simulink model "Bruening_4t_showshuffle"  (R2015a)
settings: Solver=ode4  SolverMode=MultiTasking  StartTime=0.0  StopTime=inf  FixedStep=BKIN_STEP_TIME  RelTol=1e-3
StartFcn:
  |  warndlg('Dexterit-E models cannot run under simulation. Please compile your model and run it from within Dexterit-E.');set_param(bdroot,'SimulationCommand','stop')
model workspace (MAT data in the model file):
  BKIN_STEP_TIME = 0.00025
  col_x = 1
  col_y = 2
  E_TARGET_ON = 3
  E_HOLD_AT_TARGET = 5
  LOGICAL_RADIUS = 4
  START_TARGET_COL = 1
  END_TARGET_COL = 2
  ROTATION_CENTER = 5
  WAIT_AT_1stTARGET_COL = 7
  MAXREACHTIME_COL = 8
  DELAY_POSTTRIAL_COL = 9
  E_STAY_CENTER = 2
  VISUAL_RADIUS = 3
  COLOR = 5
  ALTCOLOR = 6
  STROKECOLOUR = 7
  STROKEWIDTH = 9
  TARGET_EGG = 6
  LABEL_TEXT = 12
  LABEL_COLOUR = 13
  LABEL_HEIGHT = 14
  TEXT_DISPLAY_TARGET = 10
  ALTSTROKECOLOUR = 8
  SEGMENT_COUNT = 11
  E_TARGET_MISS = 6
  END_X = 10
  END_Y = 11
  E_LEFT_RING = 4
  E_START_BLOCK = 10
  BKIN_KINEMATIC_FRAME_SIZE = 400
  E_NO_EVENT = 1
  TARGET_IN_USE = 3
  R_PROB = 4
  E_R_TARG1 = 7
  E_M_TARG1 = 12
  E_R_TARG2 = 8
  E_M_TARG2 = 13
  E_R_TARG3 = 9
  E_M_TARG3 = 14
  E_R_TARG4 = 11
  E_M_TARG4 = 15
  WAIT_TIME = 12
  TONE_DURATION = 13
  FLASH_INTER = 14
  FLASH_NUM = 15
  BREAK_T1 = 16
  BREAK_T2 = 17
  ALTVISUAL_RADIUS = 15
  ALTCOLOR2 = 16
undefined symbols (not defined in the file or in its folder): slselsubs
libraries: Video x15, simulink x12, xpcrtudplib x12, xpcutilitieslib x10, xpcobsoletelib x8, ethercat x2, General x2, slrtlib x2, KINARM_general x1
(part 2 of 6)

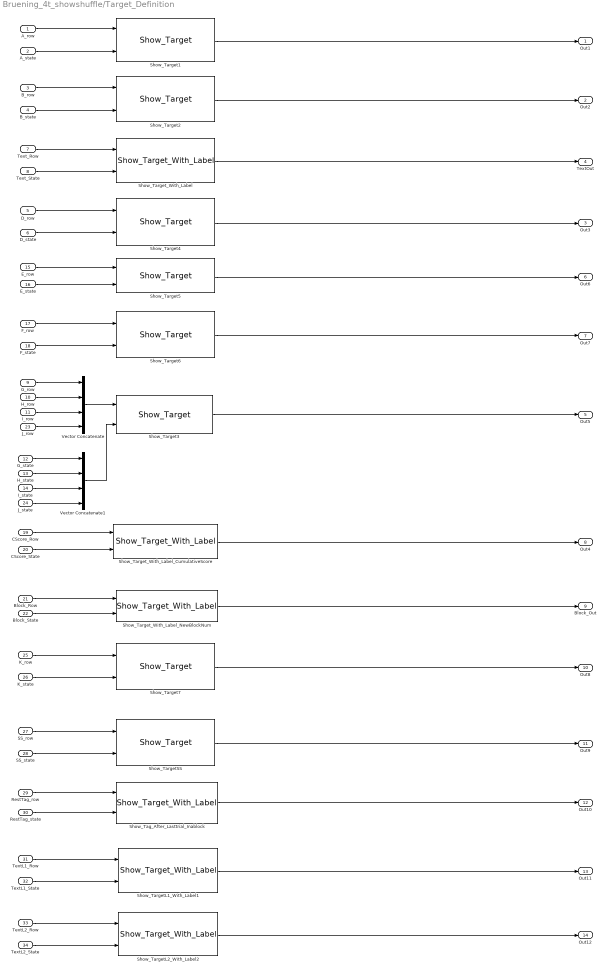
== system Bruening_4t_showshuffle/Target_Definition  ==
  A_row : Inport
  A_state : Inport  Port=2
  B_row : Inport  Port=3
  B_state : Inport  Port=4
  D_row : Inport  Port=5
  D_state : Inport  Port=6
  Text_Row : Inport  Port=7
  Text_State : Inport  Port=8
  G_row : Inport  Port=9
  H_row : Inport  Port=10
  I_row : Inport  Port=11
  G_state : Inport  Port=12
  H_state : Inport  Port=13
  I_state : Inport  Port=14
  E_row : Inport  Port=15
  E_state : Inport  Port=16
  F_row : Inport  Port=17
  F_state : Inport  Port=18
  CScore_Row : Inport  Port=19
  CScore_State : Inport  Port=20
  Block_Row : Inport  Port=21
  Block_State : Inport  Port=22
  J_row : Inport  Port=23
  J_state : Inport  Port=24
  K_row : Inport  Port=25
  K_state : Inport  Port=26
  SS_row : Inport  Port=27
  SS_state : Inport  Port=28
  RestTag_row : Inport  Port=29
  RestTag_state : Inport  Port=30
  TextL1_Row : Inport  Port=31
  TextL1_State : Inport  Port=32
  TextL2_Row : Inport  Port=33
  TextL2_State : Inport  Port=34
  Show_Tag_After_Lasttrial_Inablock : Video/Show_Target_With_Label  target_type=Circle  num_states=1  attribcol1=[0 5 0 VISUAL_RADIUS LABEL_TEXT LABEL_COLOUR LABEL_HEIGHT]  attribcol2=[6 6 0 3 0 0 0]  attribcol3=[0 0 0 0 0 0 0]  attribcol4=[0 0 0 0 0 0 0]  attribcol5=[0 0 24 0 0 0 0]  stateindices_padding=[0 0 0 0;0 0 0 0;0 0 0 0;0 0 0 0;0 0 0 0]  source=dialog  opacity=100  target_display=Both subject and operator displays
  Show_Target1 : Video/Show_Target  target_type=Circle  num_states=2  attribcol1=[COLOR 0 0 VISUAL_RADIUS]  attribcol2=[ALTCOLOR 0 0 VISUAL_RADIUS]  attribcol3=[0 0 0 0]  attribcol4=[0 0 0 0]  attribcol5=[0 0 24 0]  stateindices_padding=[0 0 0 0 0 0 0;0 0 0 0 0 0 0;0 0 0 0 0 0 0;0 0 0 0 0 0 0;0 0 0 0 0 0 0]  source=dialog  opacity=100  target_display=Both subject and operator displays  num_col=4
  Show_Target2 : Video/Show_Target  target_type=Circle  num_states=2  attribcol1=[COLOR STROKECOLOUR STROKEWIDTH VISUAL_RADIUS]  attribcol2=[COLOR ALTSTROKECOLOUR STROKEWIDTH VISUAL_RADIUS]  attribcol3=[0 0 0 0]  attribcol4=[0 0 0 0]  attribcol5=[0 0 24 0]  stateindices_padding=[0 0 0 0 0 0 0;0 0 0 0 0 0 0;0 0 0 0 0 0 0;0 0 0 0 0 0 0;0 0 0 0 0 0 0]  source=dialog  opacity=100  target_display=Both subject and operator displays  num_col=4
  Show_Target3 : Video/Show_Target  target_type=Line  num_states=2  attribcol1=[0 STROKECOLOUR STROKEWIDTH END_X END_Y]  attribcol2=[0 ALTSTROKECOLOUR STROKEWIDTH END_X END_Y]  attribcol3=[0 0 0 0 0]  attribcol4=[0 0 0 0 0]  attribcol5=[0 0 24 0 0]  stateindices_padding=[0 0 0 0 0 0;0 0 0 0 0 0;0 0 0 0 0 0;0 0 0 0 0 0;0 0 0 0 0 0]  source=dialog  opacity=100  target_display=Both subject and operator displays  num_col=5
  Show_Target4 : Video/Show_Target  target_type=Circle  num_states=3  attribcol1=[COLOR STROKECOLOUR STROKEWIDTH VISUAL_RADIUS]  attribcol2=[ALTCOLOR STROKECOLOUR STROKEWIDTH ALTVISUAL_RADIUS]  attribcol3=[ALTCOLOR2 STROKECOLOUR STROKEWIDTH VISUAL_RADIUS]  attribcol4=[0 0 0 0]  attribcol5=[0 0 24 0]  stateindices_padding=[0 0 0 0 0 0 0;0 0 0 0 0 0 0;0 0 0 0 0 0 0;0 0 0 0 0 0 0;0 0 0 0 0 0 0]  source=dialog  opacity=100  target_display=Both subject and operator displays  num_col=4
  Show_Target5 : Video/Show_Target  target_type=Circle  num_states=3  attribcol1=[COLOR STROKECOLOUR STROKEWIDTH VISUAL_RADIUS]  attribcol2=[ALTCOLOR ALTSTROKECOLOUR STROKEWIDTH ALTVISUAL_RADIUS]  attribcol3=[ALTCOLOR2 STROKECOLOUR STROKEWIDTH VISUAL_RADIUS]  attribcol4=[0 0 0 0]  attribcol5=[0 0 24 0]  stateindices_padding=[0 0 0 0 0 0 0;0 0 0 0 0 0 0;0 0 0 0 0 0 0;0 0 0 0 0 0 0;0 0 0 0 0 0 0]  source=dialog  opacity=100  target_display=Both subject and operator displays  num_col=4
  Show_Target6 : Video/Show_Target  target_type=Circle  num_states=3  attribcol1=[COLOR STROKECOLOUR STROKEWIDTH VISUAL_RADIUS]  attribcol2=[ALTCOLOR ALTSTROKECOLOUR STROKEWIDTH ALTVISUAL_RADIUS]  attribcol3=[ALTCOLOR2 STROKECOLOUR STROKEWIDTH VISUAL_RADIUS]  attribcol4=[0 0 0 0]  attribcol5=[0 0 24 0]  stateindices_padding=[0 0 0 0 0 0 0;0 0 0 0 0 0 0;0 0 0 0 0 0 0;0 0 0 0 0 0 0;0 0 0 0 0 0 0]  source=dialog  opacity=100  target_display=Both subject and operator displays  num_col=4
  Show_Target7 : Video/Show_Target  target_type=Circle  num_states=3  attribcol1=[COLOR STROKECOLOUR STROKEWIDTH VISUAL_RADIUS]  attribcol2=[ALTCOLOR ALTSTROKECOLOUR STROKEWIDTH ALTVISUAL_RADIUS]  attribcol3=[ALTCOLOR2 STROKECOLOUR STROKEWIDTH VISUAL_RADIUS]  attribcol4=[0 0 0 0]  attribcol5=[0 0 24 0]  stateindices_padding=[0 0 0 0 0 0 0;0 0 0 0 0 0 0;0 0 0 0 0 0 0;0 0 0 0 0 0 0;0 0 0 0 0 0 0]  source=dialog  opacity=100  target_display=Both subject and operator displays  num_col=4
  Show_TargetL1_With_Label1 : Video/Show_Target_With_Label  target_type=Circle  num_states=1  attribcol1=[0 5 0 VISUAL_RADIUS LABEL_TEXT LABEL_COLOUR LABEL_HEIGHT]  attribcol2=[0 6 0 VISUAL_RADIUS LABEL_TEXT LABEL_COLOUR LABEL_HEIGHT]  attribcol3=[0 0 0 0 0 0 0]  attribcol4=[0 0 0 0 0 0 0]  attribcol5=[0 0 24 0 0 0 0]  stateindices_padding=[0 0 0 0;0 0 0 0;0 0 0 0;0 0 0 0;0 0 0 0]  source=dialog  opacity=100  target_display=Both subject and operator displays
  Show_TargetL2_With_Label2 : Video/Show_Target_With_Label  target_type=Circle  num_states=1  attribcol1=[0 5 0 VISUAL_RADIUS LABEL_TEXT LABEL_COLOUR LABEL_HEIGHT]  attribcol2=[0 6 0 VISUAL_RADIUS LABEL_TEXT LABEL_COLOUR LABEL_HEIGHT]  attribcol3=[0 0 0 0 0 0 0]  attribcol4=[0 0 0 0 0 0 0]  attribcol5=[0 0 24 0 0 0 0]  stateindices_padding=[0 0 0 0;0 0 0 0;0 0 0 0;0 0 0 0;0 0 0 0]  source=dialog  opacity=100  target_display=Both subject and operator displays
  Show_TargetSS : Video/Show_Target  target_type=Circle  num_states=2  attribcol1=[COLOR STROKECOLOUR STROKEWIDTH VISUAL_RADIUS]  attribcol2=[ALTCOLOR ALTSTROKECOLOUR STROKEWIDTH VISUAL_RADIUS]  attribcol3=[0 0 0 0]  attribcol4=[0 0 0 0]  attribcol5=[0 0 24 0]  stateindices_padding=[0 0 0 0 0 0 0;0 0 0 0 0 0 0;0 0 0 0 0 0 0;0 0 0 0 0 0 0;0 0 0 0 0 0 0]  source=dialog  opacity=100  target_display=Both subject and operator displays  num_col=4
  Show_Target_With_Label : Video/Show_Target_With_Label  target_type=Circle  num_states=1  attribcol1=[0 5 0 VISUAL_RADIUS LABEL_TEXT LABEL_COLOUR LABEL_HEIGHT]  attribcol2=[0 6 0 VISUAL_RADIUS LABEL_TEXT LABEL_COLOUR LABEL_HEIGHT]  attribcol3=[0 0 0 0 0 0 0]  attribcol4=[0 0 0 0 0 0 0]  attribcol5=[0 0 24 0 0 0 0]  stateindices_padding=[0 0 0 0;0 0 0 0;0 0 0 0;0 0 0 0;0 0 0 0]  source=dialog  opacity=100  target_display=Both subject and operator displays
  Show_Target_With_Label_CumulativeScore : Video/Show_Target_With_Label  target_type=Circle  num_states=1  attribcol1=[0 5 0 VISUAL_RADIUS LABEL_TEXT LABEL_COLOUR LABEL_HEIGHT]  attribcol2=[6 6 0 3 0 0 0]  attribcol3=[0 0 0 0 0 0 0]  attribcol4=[0 0 0 0 0 0 0]  attribcol5=[0 0 24 0 0 0 0]  stateindices_padding=[0 0 0 0;0 0 0 0;0 0 0 0;0 0 0 0;0 0 0 0]  source=dialog  opacity=100  target_display=Both subject and operator displays
  Show_Target_With_Label_NewBlockNum : Video/Show_Target_With_Label  target_type=Circle  num_states=1  attribcol1=[0 5 0 VISUAL_RADIUS LABEL_TEXT LABEL_COLOUR LABEL_HEIGHT]  attribcol2=[6 6 0 3 0 0 0]  attribcol3=[0 0 0 0 0 0 0]  attribcol4=[0 0 0 0 0 0 0]  attribcol5=[0 0 24 0 0 0 0]  stateindices_padding=[0 0 0 0;0 0 0 0;0 0 0 0;0 0 0 0;0 0 0 0]  source=dialog  opacity=100  target_display=Both subject and operator displays
  Vector Concatenate : Concatenate  NumInputs=4  Mode=Multidimensional array
  Vector Concatenate1 : Concatenate  NumInputs=4  Mode=Multidimensional array
  Out1 : Outport
  Out2 : Outport  Port=2
  Out3 : Outport  Port=3
  TextOut : Outport  Port=4
  Out5 : Outport  Port=5
  Out6 : Outport  Port=6
  Out7 : Outport  Port=7
  Out4 : Outport  Port=8
  Block_Out : Outport  Port=9
  Out8 : Outport  Port=10
  Out9 : Outport  Port=11
  Out10 : Outport  Port=12
  Out11 : Outport  Port=13
  Out12 : Outport  Port=14
  wires:
  Show_Target1/1 -> Out1/1
  A_state/1 -> Show_Target1/2
  A_row/1 -> Show_Target1/1
  Text_Row/1 -> Show_Target_With_Label/1
  Text_State/1 -> Show_Target_With_Label/2
  Show_Target_With_Label/1 -> TextOut/1
  G_row/1 -> Vector Concatenate/1
  H_row/1 -> Vector Concatenate/2
  I_row/1 -> Vector Concatenate/3
  G_state/1 -> Vector Concatenate1/1
  H_state/1 -> Vector Concatenate1/2
  I_state/1 -> Vector Concatenate1/3
  Vector Concatenate/1 -> Show_Target3/1
  Vector Concatenate1/1 -> Show_Target3/2
  Show_Target3/1 -> Out5/1
  E_row/1 -> Show_Target5/1
  E_state/1 -> Show_Target5/2
  F_row/1 -> Show_Target6/1
  Show_Target5/1 -> Out6/1
  Show_Target6/1 -> Out7/1
  CScore_Row/1 -> Show_Target_With_Label_CumulativeScore/1
  CScore_State/1 -> Show_Target_With_Label_CumulativeScore/2
  Show_Target_With_Label_CumulativeScore/1 -> Out4/1
  Block_Row/1 -> Show_Target_With_Label_NewBlockNum/1
  Block_State/1 -> Show_Target_With_Label_NewBlockNum/2
  Show_Target_With_Label_NewBlockNum/1 -> Block_Out/1
  B_row/1 -> Show_Target2/1
  B_state/1 -> Show_Target2/2
  Show_Target2/1 -> Out2/1
  D_state/1 -> Show_Target4/2
  Show_Target4/1 -> Out3/1
  J_row/1 -> Vector Concatenate/4
  D_row/1 -> Show_Target4/1
  F_state/1 -> Show_Target6/2
  J_state/1 -> Vector Concatenate1/4
  Show_Target7/1 -> Out8/1
  K_row/1 -> Show_Target7/1
  K_state/1 -> Show_Target7/2
  SS_row/1 -> Show_TargetSS/1
  SS_state/1 -> Show_TargetSS/2
  Show_TargetSS/1 -> Out9/1
  Show_Tag_After_Lasttrial_Inablock/1 -> Out10/1
  RestTag_row/1 -> Show_Tag_After_Lasttrial_Inablock/1
  RestTag_state/1 -> Show_Tag_After_Lasttrial_Inablock/2
  TextL1_Row/1 -> Show_TargetL1_With_Label1/1
  TextL1_State/1 -> Show_TargetL1_With_Label1/2
  TextL2_State/1 -> Show_TargetL2_With_Label2/2
  TextL2_Row/1 -> Show_TargetL2_With_Label2/1
  Show_TargetL2_With_Label2/1 -> Out12/1
  Show_TargetL1_With_Label1/1 -> Out11/1

== system Bruening_4t_showshuffle/DataLogging/Create Analog Inputs Subsystem ==
  In1 : Inport
  Analog Data : DataTypeConversion  SaturateOnIntegerOverflow=on  RndMeth=Zero
  Analog Data Width : DataTypeConversion  SaturateOnIntegerOverflow=on  RndMeth=Zero
  Mux2 : Mux  Inputs=2
  Not Logging Analog Inputs : Constant
  Rate Transition : RateTransition
  Rate Transition1 : RateTransition
  Subtract : Sum  Inputs=-+
  Width : Width
  Out1 : Outport
  wires:
  Mux2/1 -> Out1/1
  In1/1 -> Analog Data/1, Width/1
  Subtract/1 -> Analog Data Width/1
  Not Logging Analog Inputs/1 -> Subtract/1
  Analog Data Width/1 -> Rate Transition/1
  Width/1 -> Subtract/2
  Analog Data/1 -> Rate Transition1/1
  Rate Transition/1 -> Mux2/1
  Rate Transition1/1 -> Mux2/2

== system Bruening_4t_showshuffle/DataLogging/Create Custom Data Subsystem ==
  Custom Data1 : DataTypeConversion  SaturateOnIntegerOverflow=on  RndMeth=Zero
  Mux1 : Mux  Inputs=3
  Mux6 : Mux  Inputs=2
  Rate Transition : RateTransition
  Width : Width
  custom_version : Constant  Value=5  OutDataTypeStr=double
  Out1 : Outport
  wires:
  Mux6/1 -> Out1/1
  Mux1/1 -> Width/1, Mux6/2
  Width/1 -> Mux6/1
  custom_version/1 -> Mux1/1
  [status_data] -> Custom Data1/1
  [encoderDeltas] -> Rate Transition/1
  Custom Data1/1 -> Mux1/2
  Rate Transition/1 -> Mux1/3

== system Bruening_4t_showshuffle/DataLogging/Create Event Codes Subsystem ==
  In1 : Inport
  Event Codes : DataTypeConversion  SaturateOnIntegerOverflow=on  RndMeth=Zero
  Mux4 : Mux  Inputs=2
  Not Logging Event Codes : Constant  Value=0
  Number of Event Codes : DataTypeConversion  SaturateOnIntegerOverflow=on  RndMeth=Zero
  Subtract : Sum  Inputs=-+
  Width : Width
  Out1 : Outport
  wires:
  Mux4/1 -> Out1/1
  In1/1 -> Event Codes/1, Width/1
  Not Logging Event Codes/1 -> Subtract/1
  Subtract/1 -> Number of Event Codes/1
  Width/1 -> Subtract/2
  Number of Event Codes/1 -> Mux4/1
  Event Codes/1 -> Mux4/2

== system Bruening_4t_showshuffle/DataLogging/Create KINARM Data Subsystem ==
  Arm Kinematics : DataTypeConversion  SaturateOnIntegerOverflow=on  RndMeth=Zero
  Bus Selector : BusSelector  OutputSignals=Robot1.a1_link_angles,Robot1.a1_link_velocities,Robot1.a1_link_accelerations,Robot1.a1_hand_position,Robot1.a1_motor_torque_command,Robot1.a1_force_sensor_force_xyz,Robot1.a1_force_sensor_torque_xyz,Robot1.a1_force_sensor_timestamp,Robot1.a1_ecatRecordedMotorTorques,Robot2.a2_link_angles,Robot2.a2_link_velocities,Robot2.a2_link_accelerations,Robot2.a2_hand_position,Robot2.a2_motor_torque_command,Robot2.a2_force_sensor_force_xyz,Robot2.a2_force_sensor_torque_xyz,Robot2.a2_force_sensor_timestamp,Robot2.a2_ecatRecordedMotorTorques  OutputAsBus=on
  Bus Selector1 : BusSelector  OutputSignals=Robot1.a1_motor_status,Robot2.a2_motor_status,Robot1.a1_ecatCurrentLimitEnabled,Robot2.a2_ecatCurrentLimitEnabled  OutputAsBus=on
  Bus to Vector : BusToVector
  Bus to Vector1 : BusToVector
  Kinarm Data Width : DataTypeConversion  SaturateOnIntegerOverflow=on  RndMeth=Zero
  Mux : Mux  Inputs=3
  Mux1 : Mux  Inputs=2
  Mux3 : Mux
  Rate Transition{,1..3} (4 alike) : RateTransition
  Width : Width
  bitfield : MATLAB Function  TreatAsAtomicUnit=on
  touint : DataTypeConversion  OutDataTypeStr=uint32  SaturateOnIntegerOverflow=on  RndMeth=Zero
  touint1 : DataTypeConversion  OutDataTypeStr=double  SaturateOnIntegerOverflow=on  RndMeth=Zero
  Out1 : Outport
  wires:
  Mux1/1 -> Out1/1
  Rate Transition/1 -> Mux3/1
  Mux3/1 -> Width/1, Arm Kinematics/1
  Bus Selector/1 -> Bus to Vector/1
  Kinarm Data Width/1 -> Mux1/1
  Width/1 -> Kinarm Data Width/1
  Arm Kinematics/1 -> Mux1/2
  Rate Transition2/1 -> Mux3/2
  Rate Transition3/1 -> Mux3/3
  [ForcePlateData] -> Rate Transition3/1
  [Gaze_Global] -> Mux/1
  Mux/1 -> Rate Transition2/1
  [Gaze_Event_Info] -> Mux/3
  [Gaze_pupil_area] -> Mux/2
  [KINdata_bus] -> Bus Selector/1
  Bus to Vector/1 -> Rate Transition/1
  [KINdata_bus] -> Bus Selector1/1
  Bus Selector1/1 -> Bus to Vector1/1
  Bus to Vector1/1 -> touint/1
  bitfield/1(bitfield) -> Rate Transition1/1
  Rate Transition1/1 -> touint1/1
  touint/1 -> bitfield/1(motorStatus)
  touint1/1 -> Mux3/4

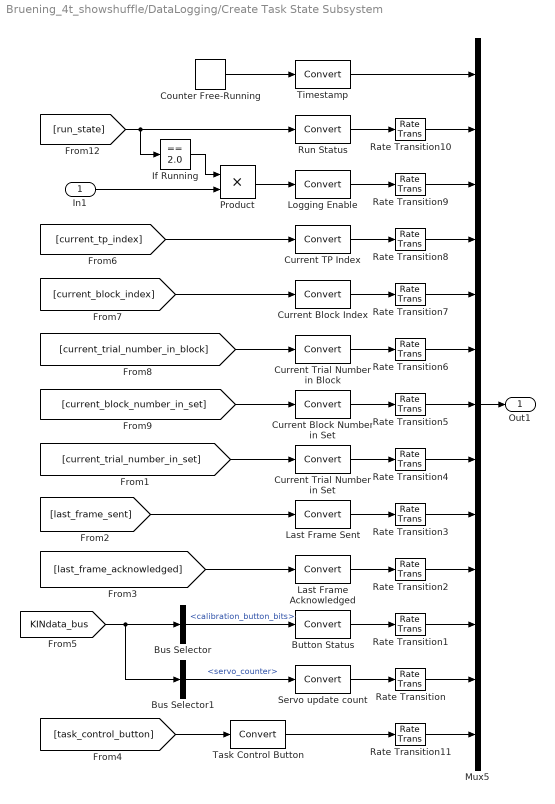
== system Bruening_4t_showshuffle/DataLogging/Create Task State Subsystem ==
  In1 : Inport
  Bus Selector : BusSelector  OutputSignals=KINDataGeneral.calibration_button_bits
  Bus Selector1 : BusSelector  OutputSignals=KINDataGeneral.servo_counter
  Button Status : DataTypeConversion  SaturateOnIntegerOverflow=on  RndMeth=Zero
  Counter Free-Running : simulink/Sources/Counter Free-Running  NumBits=32  tsamp=-1
  Current Block Index : DataTypeConversion  SaturateOnIntegerOverflow=on  RndMeth=Zero
  Current Block Number in Set : DataTypeConversion  SaturateOnIntegerOverflow=on  RndMeth=Zero
  Current TP Index : DataTypeConversion  SaturateOnIntegerOverflow=on  RndMeth=Zero
  Current Trial Number in Block : DataTypeConversion  SaturateOnIntegerOverflow=on  RndMeth=Zero
  Current Trial Number in Set : DataTypeConversion  SaturateOnIntegerOverflow=on  RndMeth=Zero
  If Running : simulink/Logic and Bit Operations/Compare To Constant  relop===  const=2.0  OutDataTypeStr=uint8  ZeroCross=off
  Last Frame Acknowledged : DataTypeConversion  SaturateOnIntegerOverflow=on  RndMeth=Zero
  Last Frame Sent : DataTypeConversion  SaturateOnIntegerOverflow=on  RndMeth=Zero
  Logging Enable : DataTypeConversion  SaturateOnIntegerOverflow=on  RndMeth=Zero
  Mux5 : Mux  Inputs=13
  Product : Product  RndMeth=Zero
  Rate Transition{,1..11} (12 alike) : RateTransition
  Run Status : DataTypeConversion  SaturateOnIntegerOverflow=on  RndMeth=Zero
  Servo update count : DataTypeConversion  SaturateOnIntegerOverflow=on  RndMeth=Zero
  Task Control Button : DataTypeConversion  SaturateOnIntegerOverflow=on  RndMeth=Zero
  Timestamp : DataTypeConversion  SaturateOnIntegerOverflow=on  RndMeth=Zero
  Out1 : Outport
  wires:
  Task Control Button/1 -> Rate Transition11/1
  [task_control_button] -> Task Control Button/1
  Button Status/1 -> Rate Transition1/1
  [last_frame_acknowledged] -> Last Frame Acknowledged/1
  [last_frame_sent] -> Last Frame Sent/1
  Last Frame Acknowledged/1 -> Rate Transition2/1
  Last Frame Sent/1 -> Rate Transition3/1
  Mux5/1 -> Out1/1
  In1/1 -> Product/2
  Current Trial Number in Set/1 -> Rate Transition4/1
  Current Block Number in Set/1 -> Rate Transition5/1
  Current Trial Number in Block/1 -> Rate Transition6/1
  Current Block Index/1 -> Rate Transition7/1
  Current TP Index/1 -> Rate Transition8/1
  Logging Enable/1 -> Rate Transition9/1
  Run Status/1 -> Rate Transition10/1
  Timestamp/1 -> Mux5/1
  [current_trial_number_in_set] -> Current Trial Number in Set/1
  [current_block_number_in_set] -> Current Block Number in Set/1
  [current_trial_number_in_block] -> Current Trial Number in Block/1
  [current_block_index] -> Current Block Index/1
  [current_tp_index] -> Current TP Index/1
  If Running/1 -> Product/1
  Counter Free-Running/1 -> Timestamp/1
  [run_state] -> If Running/1, Run Status/1
  Product/1 -> Logging Enable/1
  Servo update count/1 -> Rate Transition/1
  Bus Selector1/1 -> Servo update count/1  "<servo_counter>"
  Rate Transition/1 -> Mux5/12
  Rate Transition1/1 -> Mux5/11
  Rate Transition2/1 -> Mux5/10
  Rate Transition3/1 -> Mux5/9
  Rate Transition4/1 -> Mux5/8
  Rate Transition5/1 -> Mux5/7
  Rate Transition6/1 -> Mux5/6
  Rate Transition7/1 -> Mux5/5
  Rate Transition8/1 -> Mux5/4
  Rate Transition9/1 -> Mux5/3
  Rate Transition10/1 -> Mux5/2
  [KINdata_bus] -> Bus Selector/1, Bus Selector1/1
  Bus Selector/1 -> Button Status/1  "<calibration_button_bits>"
  Rate Transition11/1 -> Mux5/13

== system Bruening_4t_showshuffle/DataLogging/Keep alive ==
  note: Every 100ms this sends out a message that
      | DexDisplay should get and replay to Dex.
      | That is how Dex can tell if DexDisplay is blocked by a firewall.
  Pack : xpcobsoletelib/Utilities/Pack   datatypes={'double'}  byteAlign=1
  Send : xpcrtudplib/Legacy UDP/Send   ipAddress=192.168.0.1  ipPort=50010  localPort=-1  vblLen=off  sampletime=0.1
  const : Constant  Value=[1 1 1 1 1]  OutDataTypeStr=double
  wires:
  const/1 -> Pack/1
  Pack/1 -> Send/1

== system Bruening_4t_showshuffle/DataLogging/Network Transfer Subsystem ==
  note: This subsystem controls the assembly, buffering, and sending of data packets, as well as the receipt of acknowledgements (ACKs). The data packing subsystem packs
      | together multiple data frames, and when its strobe output is set high the send control machine uses this data to create a new packet in its internal ring buffer. Each
      | packet consists of a tracking number, one or more data frames, and a trailing 0. The latter guarantees that the end of the data can be determined by a 0 found in
      | place of a data frame timestamp.
      |
      | The send control machine will send the next packet in its buffer after an ACK for the previous one is received. If it  will resend a packet if it has not received an ACK
      | after a fixed time, and repeat the send for every elapse of that time. Currently up to 5000 packets - a minimum of 5 seconds and a maximum of 30 seconds of data,
      | depending on frame size - are buffered.
  note: This Send control system is basically trying to make a reliable system out of UDP.
      | 1. Packets are built with one or more kinematics frames of data
      | 2. The packets are added to an internal queue of 50k potential packets
      | 3. A packet is sent to Dex
      | 4. Dex sends an ACK for the given packet
      | 5. The cycle starts again.
      |
      | When ACKs are not received then we attempt to resend the packet.
  data_frame : Inport
  global clock : Inport  Port=2
  run_status : Inport  Port=3
  Data Packing Subsystem : Subsystem  TreatAsAtomicUnit=on  SystemSampleTime=0.001
  Data Type Conversion2 : DataTypeConversion
  Mux1 : Mux  Inputs=3
  Queue Size : DataTypeConversion  OutDataTypeStr=double  SaturateOnIntegerOverflow=on  RndMeth=Zero
  Send Control Machine : Stateflow chart  TreatAsAtomicUnit=on
  Task Clock : DiscretePulseGenerator  PulseType=Time based  Period=BKIN_STEP_TIME * 2  PulseWidth=50  SampleTime=0.0005
  Terminator : Terminator
  Terminator1 : Terminator
  Terminator2 : Terminator
  Total Timeouts : DataTypeConversion  OutDataTypeStr=double  SaturateOnIntegerOverflow=on  RndMeth=Zero
  UDP Receiver : Subsystem
  UDP Send Subsystem : Subsystem  TreatAsAtomicUnit=on
  force strobe1 : MATLAB Function  TreatAsAtomicUnit=on  SystemSampleTime=0.0005
  max_packet_id : Constant  Value=8000000  OutDataTypeStr=uint32
  runID : Constant  Value=0  OutDataTypeStr=double
  wires:
  data_frame/1 -> Data Packing Subsystem/1(data_frame)
  Send Control Machine/2(data_out) -> UDP Send Subsystem/1(packet_data)
  Send Control Machine/5(e_send()) -> UDP Send Subsystem/Trigger
  Data Packing Subsystem/1(daq_packet_strobe) -> force strobe1/1(strobe)
  Send Control Machine/3(queue_size) -> Queue Size/1
  Send Control Machine/4(total_timeouts) -> Total Timeouts/1
  Mux1/1 -> Send Control Machine/Trigger
  Data Packing Subsystem/2(packed_data) -> Send Control Machine/1(data_in)
  UDP Send Subsystem/1(total_packets_sent) -> Terminator/1  "packet_counter"
  max_packet_id/1 -> Send Control Machine/3(max_packet_id)
  runID/1 -> Data Type Conversion2/1
  Data Type Conversion2/1 -> Send Control Machine/4(runID)
  force strobe1/1(strobe_out) -> Mux1/1
  Queue Size/1 -> Terminator1/1  "queue_size"
  Total Timeouts/1 -> Terminator2/1  "timeouts"
  global clock/1 -> Mux1/2
  Task Clock/1 -> Mux1/3
  UDP Receiver/1(ACK_ID) -> Send Control Machine/2(ack_packet_index)
  Send Control Machine/1(resetUDP) -> [reset_UDP]  "Trigger"
  [reset_UDP] -> UDP Receiver/1(Trigger UDP reset)
  run_status/1 -> Send Control Machine/5(exam_is_running)

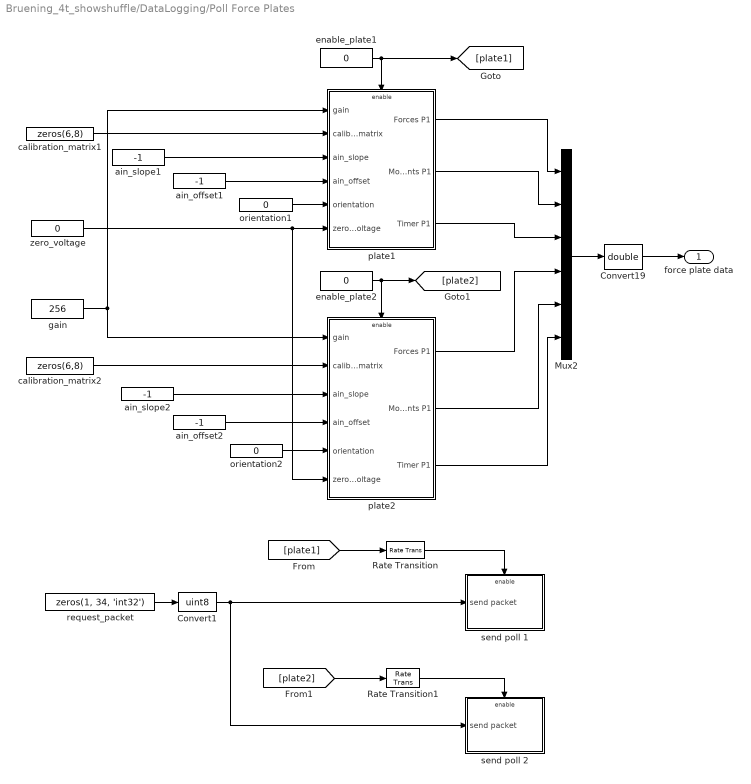
== system Bruening_4t_showshuffle/DataLogging/Poll Force Plates ==
  Convert1 : DataTypeConversion  OutDataTypeStr=uint8
  Convert19 : DataTypeConversion  OutDataTypeStr=double
  Mux2 : Mux  Inputs=6
  Rate Transition : RateTransition  OutPortSampleTime=0.0005
  Rate Transition1 : RateTransition  OutPortSampleTime=0.0005
  ain_offset1 : Constant  Value=-1
  ain_offset2 : Constant  Value=-1
  ain_slope1 : Constant  Value=-1
  ain_slope2 : Constant  Value=-1
  calibration_matrix1 : Constant  Value=zeros(6,8)
  calibration_matrix2 : Constant  Value=zeros(6,8)
  enable_plate1 : Constant  Value=0  SampleTime=BKIN_STEP_TIME
  enable_plate2 : Constant  Value=0  SampleTime=BKIN_STEP_TIME
  gain : Constant  Value=256
  orientation1 : Constant  Value=0
  orientation2 : Constant  Value=0
  plate1 : Subsystem
  plate2 : Subsystem
  request_packet : Constant  Value=zeros(1, 34, 'int32')  SampleTime=BKIN_STEP_TIME
  send poll 1 : Subsystem
  send poll 2 : Subsystem
  zero_voltage : Constant  Value=0
  force plate data : Outport
  wires:
  gain/1 -> plate2/1(gain), plate1/1(gain)
  plate1/1(Forces P1) -> Mux2/1
  plate1/2(Moments P1) -> Mux2/2
  plate1/3(Timer P1) -> Mux2/3
  plate2/1(Forces P1) -> Mux2/4
  plate2/2(Moments P1) -> Mux2/5
  plate2/3(Timer P1) -> Mux2/6
  calibration_matrix1/1 -> plate1/2(calib_matrix)
  calibration_matrix2/1 -> plate2/2(calib_matrix)
  enable_plate1/1 -> plate1/Enable, [plate1]
  enable_plate2/1 -> plate2/Enable, [plate2]
  Mux2/1 -> Convert19/1
  ain_slope1/1 -> plate1/3(ain_slope)
  ain_offset1/1 -> plate1/4(ain_offset)
  ain_slope2/1 -> plate2/3(ain_slope)
  ain_offset2/1 -> plate2/4(ain_offset)
  orientation1/1 -> plate1/5(orientation)
  orientation2/1 -> plate2/5(orientation)
  Convert19/1 -> force plate data/1
  request_packet/1 -> Convert1/1
  zero_voltage/1 -> plate1/6(zero_voltage), plate2/6(zero_voltage)
  Convert1/1 -> send poll 1/1(send packet), send poll 2/1(send packet)
  Rate Transition1/1 -> send poll 2/Enable
  [plate1] -> Rate Transition/1
  [plate2] -> Rate Transition1/1
  Rate Transition/1 -> send poll 1/Enable

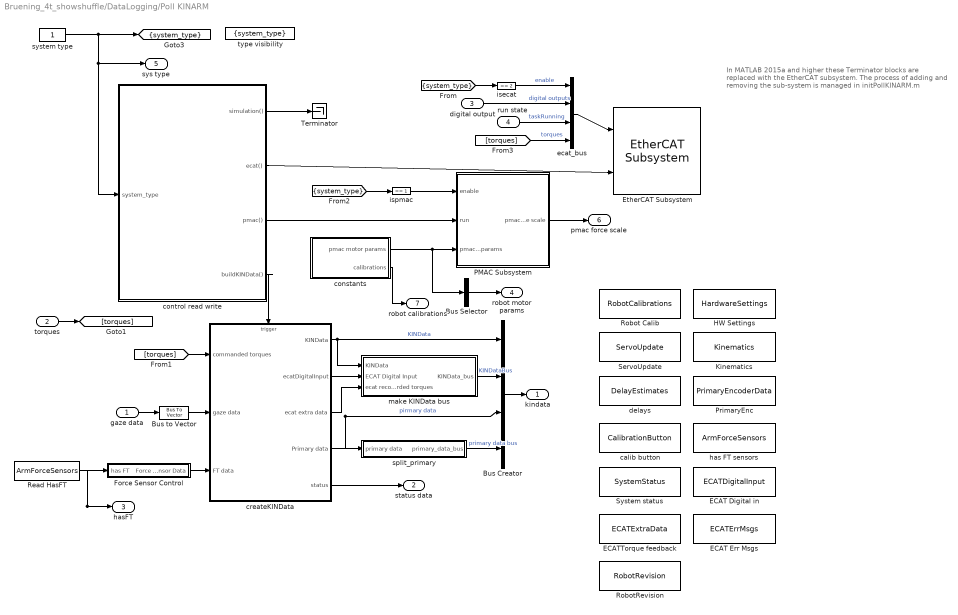
== system Bruening_4t_showshuffle/DataLogging/Poll KINARM ==
  note: In MATLAB 2015a and higher these Terminator blocks
      | are replaced with the EtherCAT subsystem. The process of
      | adding and removing the sub-system is managed in
      | initPollKINARM.m
  gaze data : Inport
  torques : Inport  Port=2
  digital output : Inport  Port=3
  run state : Inport  Port=4
  Bus Creator : BusCreator
  Bus Selector : BusSelector  OutputSignals=robot1MotorParams,robot2MotorParams  OutputAsBus=on
  Bus to Vector : BusToVector
  ECAT Digital in : DataStoreMemory  DataStoreName=ECATDigitalInput  ReadBeforeWriteMsg=error  WriteAfterWriteMsg=warning  WriteAfterReadMsg=error  InitialValue=[0, 0, 0, 0, 0, 0, 0, 0]  OutDataTypeStr=uint32
  ECAT Err Msgs : DataStoreMemory  DataStoreName=ECATErrMsgs  ReadBeforeWriteMsg=error  WriteAfterWriteMsg=warning  WriteAfterReadMsg=error  InitialValue=zeros(4, 5)  OutDataTypeStr=double
  ECATTorque feedback : DataStoreMemory  DataStoreName=ECATExtraData  ReadBeforeWriteMsg=error  WriteAfterWriteMsg=warning  WriteAfterReadMsg=error  InitialValue=[0, 0, 0, 0, 0, 0, 0, 0]  OutDataTypeStr=double
  EtherCAT Subsystem : ethercat/EtherCAT Subsystem  SystemSampleTime=BKIN_STEP_TIME
  Force Sensor Control : Subsystem  TreatAsAtomicUnit=on
      settings: RTWSystemCode=Nonreusable function  RTWFileNameOpts=Use function name
  HW Settings : DataStoreMemory  DataStoreName=HardwareSettings  ReadBeforeWriteMsg=error  WriteAfterWriteMsg=warning  WriteAfterReadMsg=error  InitialValue=zeros(24, 1)  OutDataTypeStr=double
  Kinematics : DataStoreMemory  DataStoreName=Kinematics  ReadBeforeWriteMsg=error  WriteAfterWriteMsg=warning  WriteAfterReadMsg=error  InitialValue=zeros(20, 1)  OutDataTypeStr=double
  PMAC Subsystem : Subsystem
      settings: RTWSystemCode=Nonreusable function  RTWFileNameOpts=Use function name
  PrimaryEnc : DataStoreMemory  DataStoreName=PrimaryEncoderData  ReadBeforeWriteMsg=error  WriteAfterWriteMsg=warning  WriteAfterReadMsg=error  InitialValue=zeros(12, 1)  OutDataTypeStr=double
  Read HasFT : DataStoreRead  DataStoreName=ArmForceSensors  SampleTime=BKIN_STEP_TIME
  Robot Calib : DataStoreMemory  DataStoreName=RobotCalibrations  InitialValue=zeros(16, 1)  OutDataTypeStr=double
  RobotRevision : DataStoreMemory  DataStoreName=RobotRevision  ReadBeforeWriteMsg=error  WriteAfterWriteMsg=warning  WriteAfterReadMsg=error  InitialValue=[1, 1]  OutDataTypeStr=double
  ServoUpdate : DataStoreMemory  DataStoreName=ServoUpdate  ReadBeforeWriteMsg=error  WriteAfterWriteMsg=warning  WriteAfterReadMsg=error  OutDataTypeStr=uint32
  System status : DataStoreMemory  DataStoreName=SystemStatus  ReadBeforeWriteMsg=error  WriteAfterWriteMsg=warning  WriteAfterReadMsg=error  InitialValue=zeros(1, 7)  OutDataTypeStr=uint32
  Terminator : Terminator
  calib button : DataStoreMemory  DataStoreName=CalibrationButton  ReadBeforeWriteMsg=error  WriteAfterWriteMsg=warning  WriteAfterReadMsg=error  OutDataTypeStr=uint32
  constants : Subsystem
      settings: RTWSystemCode=Nonreusable function  RTWFileNameOpts=Use function name
  control read write : Stateflow chart  TreatAsAtomicUnit=on
  createKINData : Subsystem
      settings: RTWSystemCode=Nonreusable function  RTWFileNameOpts=Use function name
  delays : DataStoreMemory  DataStoreName=DelayEstimates  ReadBeforeWriteMsg=error  WriteAfterWriteMsg=warning  WriteAfterReadMsg=error  InitialValue=zeros(4, 1)  OutDataTypeStr=double
  ecat_bus : BusCreator
  has FT sensors : DataStoreMemory  DataStoreName=ArmForceSensors  InitialValue=[0, 0]  OutDataTypeStr=double
  isecat : simulink/Logic and Bit Operations/Compare To Constant  relop===  const=2  OutDataTypeStr=boolean
  ispmac : simulink/Logic and Bit Operations/Compare To Constant  relop===  const=1  OutDataTypeStr=boolean
  make KINData bus : Subsystem
  split_primary : Subsystem
  system type : Constant
  type visibility : GotoTagVisibility  GotoTag=system_type
  kindata : Outport
  status data : Outport  Port=2
  hasFT : Outport  Port=3
  robot motor params : Outport  Port=4
  sys type : Outport  Port=5
  pmac force scale : Outport  Port=6
  robot calibrations : Outport  Port=7
  tag scope: system_type=scoped
  wires:
  Bus Selector/1 -> robot motor params/1
  Bus Creator/1 -> kindata/1
  Bus to Vector/1 -> createKINData/2(gaze data)
  constants/1(pmac motor params) -> Bus Selector/1, PMAC Subsystem/3(pmac robot params)
  createKINData/1(KINData) -> Bus Creator/1, make KINData bus/1(KINData)  "KINData"
  createKINData/4(Primary data) -> Bus Creator/3, split_primary/1(primary data)  "pirmary data"
  createKINData/5(status) -> status data/1
  gaze data/1 -> Bus to Vector/1
  Force Sensor Control/1(Force Sensor Data) -> createKINData/3(FT data)
  system type/1 -> [system_type], control read write/1(system_type), sys type/1
  control read write/1(simulation()) -> Terminator/1
  control read write/3(pmac()) -> PMAC Subsystem/2(run)
  control read write/4(buildKINData()) -> createKINData/Trigger
  [system_type] -> isecat/1
  [system_type] -> ispmac/1
  ispmac/1 -> PMAC Subsystem/1(enable)
  Read HasFT/1 -> Force Sensor Control/1(has FT), hasFT/1
  make KINData bus/1(KINData_bus) -> Bus Creator/2  "KINDataBus"
  split_primary/1(primary_data_bus) -> Bus Creator/4  "primary data bus"
  PMAC Subsystem/1(pmac force scale) -> pmac force scale/1
  constants/2(calibrations) -> robot calibrations/1
  createKINData/2(ecatDigitalInput) -> make KINData bus/2(ECAT Digital Input)
  digital output/1 -> ecat_bus/2  "digital outputs"
  run state/1 -> ecat_bus/3  "taskRunning"
  isecat/1 -> ecat_bus/1  "enable"
  torques/1 -> [torques]
  [torques] -> createKINData/1(commanded torques)
  [torques] -> ecat_bus/4  "torques"
  createKINData/3(ecat extra data) -> make KINData bus/3(ecat recorded torques)
  ecat_bus/1 -> EtherCAT Subsystem/1
  control read write/2(ecat()) -> EtherCAT Subsystem/2

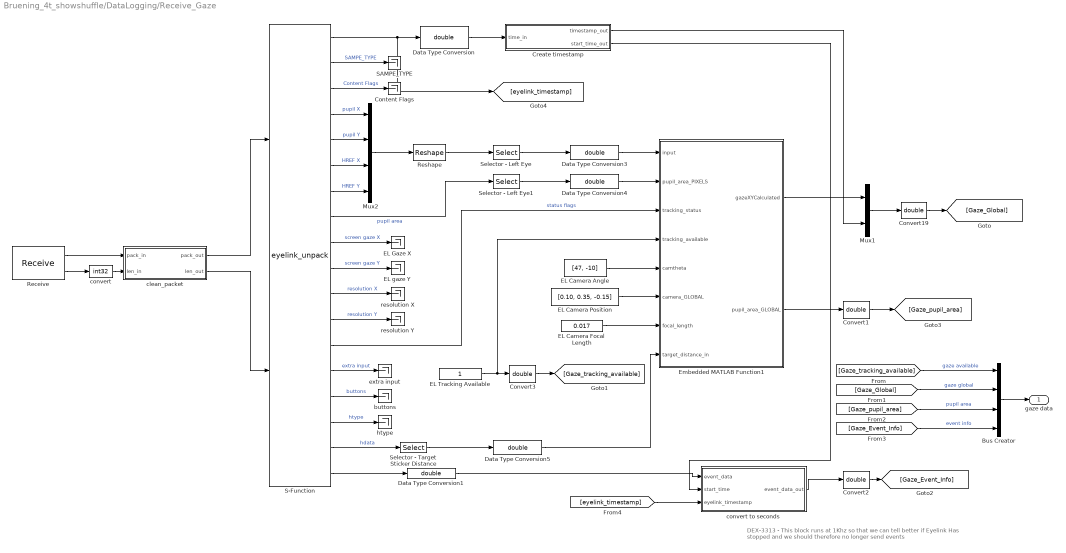
== system Bruening_4t_showshuffle/DataLogging/Receive_Gaze ==
  note: DEX-3313 - This block runs at 1Khz so that we can tell better if Eyelink
      | Has stopped and we should therefore no longer send events
  Bus Creator : BusCreator
  Content Flags : Terminator
  Convert{1..3,19} (4 alike) : DataTypeConversion  OutDataTypeStr=double
  Create timestamp : MATLAB Function  TreatAsAtomicUnit=on
  Data Type Conversion{,1,3..5} (5 alike) : DataTypeConversion  OutDataTypeStr=double
  EL Camera Angle : Constant  Value=[47, -10]  VectorParams1D=off  OutDataTypeStr=double
  EL Camera Focal Length : Constant  Value=0.017  VectorParams1D=off  OutDataTypeStr=double
  EL Camera Position : Constant  Value=[0.10, 0.35, -0.15]  VectorParams1D=off  OutDataTypeStr=double
  EL Gaze X : Terminator
  EL Tracking Available : Constant  VectorParams1D=off  OutDataTypeStr=double
  EL gaze Y : Terminator
  Embedded MATLAB Function1 : MATLAB Function  TreatAsAtomicUnit=on
  Mux1 : Mux  Inputs=2
  Mux2 : Mux
  Receive : xpcrtudplib/Legacy UDP/Receive   ipAddress=0.0.0.0  ipPort=4000  width=512  vblLen=on  sampletime=BKIN_STEP_TIME
  Reshape : Reshape  OutputDimensionality=Customize  OutputDimensions=[2,4]
  S-Function : S-Function  FunctionName=eyelink_unpack
  SAMPE_TYPE : Terminator
  Selector - Left Eye : Selector  NumberOfDimensions=2  InputPortWidth=3  IndexOptions=Index vector (dialog),Index vector (dialog)  Indices=1,-1  OutputSizes=1,1
  Selector - Left Eye1 : Selector
  Selector - Target Sticker Distance : Selector  Indices=3
  buttons : Terminator
  clean_packet : MATLAB Function  TreatAsAtomicUnit=on
  convert : DataTypeConversion  OutDataTypeStr=int32
  convert to seconds : MATLAB Function  TreatAsAtomicUnit=on
  extra input : Terminator
  htype : Terminator
  resolution X : Terminator
  resolution Y : Terminator
  gaze data : Outport
  wires:
  [eyelink_timestamp] -> convert to seconds/3(eyelink_timestamp)
  Bus Creator/1 -> gaze data/1
  [Gaze_Event_Info] -> Bus Creator/4  "event info"
  [Gaze_pupil_area] -> Bus Creator/3  "pupil area"
  [Gaze_Global] -> Bus Creator/2  "gaze global"
  [Gaze_tracking_available] -> Bus Creator/1  "gaze available"
  EL Tracking Available/1 -> Embedded MATLAB Function1/4(tracking_available), Convert3/1
  EL Camera Position/1 -> Embedded MATLAB Function1/6(camera_GLOBAL)
  EL Camera Angle/1 -> Embedded MATLAB Function1/5(camtheta)
  Selector - Target Sticker Distance/1 -> Data Type Conversion5/1
  Selector - Left Eye/1 -> Data Type Conversion3/1
  Reshape/1 -> Selector - Left Eye/1
  Mux2/1 -> Reshape/1
  S-Function/7 -> Mux2/4  "HREF Y"
  S-Function/6 -> Mux2/3  "HREF X"
  S-Function/5 -> Mux2/2  "pupil Y"
  S-Function/4 -> Mux2/1  "pupil X"
  Receive/2 -> convert/1
  S-Function/17 -> Selector - Target Sticker Distance/1  "hdata"
  S-Function/16 -> htype/1  "htype"
  S-Function/15 -> buttons/1  "buttons"
  S-Function/14 -> extra input/1  "extra input"
  S-Function/13 -> Embedded MATLAB Function1/3(tracking_status)  "status flags"
  S-Function/12 -> resolution Y/1  "resolution Y"
  S-Function/11 -> resolution X/1  "resolution X"
  S-Function/8 -> Selector - Left Eye1/1  "pupil area"
  S-Function/3 -> Content Flags/1  "Content Flags"
  S-Function/2 -> SAMPE_TYPE/1  "SAMPE_TYPE"
  S-Function/9 -> EL Gaze X/1  "screen gaze X"
  S-Function/10 -> EL gaze Y/1  "screen gaze Y"
  Mux1/1 -> Convert19/1
  Embedded MATLAB Function1/1(gazeXYCalculated) -> Mux1/1
  Create timestamp/1(timestamp_out) -> Mux1/2
  Data Type Conversion/1 -> Create timestamp/1(time_in)
  S-Function/1 -> [eyelink_timestamp], Data Type Conversion/1
  S-Function/18 -> Data Type Conversion1/1
  Data Type Conversion1/1 -> convert to seconds/1(event_data)
  convert to seconds/1(event_data_out) -> Convert2/1
  Create timestamp/2(start_time_out) -> convert to seconds/2(start_time)
  Data Type Conversion3/1 -> Embedded MATLAB Function1/1(input)
  Data Type Conversion5/1 -> Embedded MATLAB Function1/8(target_distance_in)
  Embedded MATLAB Function1/2(pupil_area_GLOBAL) -> Convert1/1
  Data Type Conversion4/1 -> Embedded MATLAB Function1/2(pupil_area_PIXELS)
  EL Camera Focal Length/1 -> Embedded MATLAB Function1/7(focal_length)
  Selector - Left Eye1/1 -> Data Type Conversion4/1
  Receive/1 -> clean_packet/1(pack_in)
  convert/1 -> clean_packet/2(len_in)
  clean_packet/1(pack_out) -> S-Function/1
  clean_packet/2(len_out) -> S-Function/2
  Convert19/1 -> [Gaze_Global]
  Convert1/1 -> [Gaze_pupil_area]
  Convert2/1 -> [Gaze_Event_Info]
  Convert3/1 -> [Gaze_tracking_available]

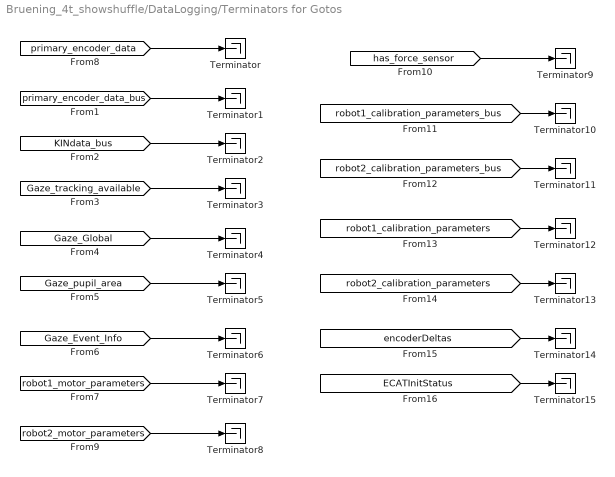
== system Bruening_4t_showshuffle/DataLogging/Terminators for Gotos ==
  Terminator{,1..15} (16 alike) : Terminator
  wires:
  [has_force_sensor] -> Terminator9/1
  [robot2_motor_parameters] -> Terminator8/1
  [robot1_motor_parameters] -> Terminator7/1
  [Gaze_Event_Info] -> Terminator6/1
  [Gaze_pupil_area] -> Terminator5/1
  [Gaze_Global] -> Terminator4/1
  [Gaze_tracking_available] -> Terminator3/1
  [KINdata_bus] -> Terminator2/1
  [primary_encoder_data_bus] -> Terminator1/1
  [primary_encoder_data] -> Terminator/1
  [robot1_calibration_parameters_bus] -> Terminator10/1
  [robot2_calibration_parameters_bus] -> Terminator11/1
  [robot1_calibration_parameters] -> Terminator12/1
  [robot2_calibration_parameters] -> Terminator13/1
  [encoderDeltas] -> Terminator14/1
  [ECATInitStatus] -> Terminator15/1

== system Bruening_4t_showshuffle/DataLogging/apply loads ==
  system_type : Inport
  torques : Inport  Port=2
  pmac force scale : Inport  Port=3
  motor params : Inport  Port=4
  Bus Selector3 : BusSelector  OutputSignals=robot1MotorParams,robot2MotorParams
  EtherCAT Apply Loads : ethercat/ECAT Apply Loads
  apply pmac loads : Subsystem
      settings: RTWSystemCode=Nonreusable function  RTWFileNameOpts=Use function name
  isecat : simulink/Logic and Bit Operations/Compare To Constant  relop===  const=2  OutDataTypeStr=boolean
  isecat1 : simulink/Logic and Bit Operations/Compare To Constant  relop===  const=1  OutDataTypeStr=boolean
  wires:
  Bus Selector3/2 -> apply pmac loads/4(Robot 2 motor parms)  "<robot2MotorParams>"
  Bus Selector3/1 -> apply pmac loads/3(Robot 1 motor parms)  "<robot1MotorParams>"
  pmac force scale/1 -> apply pmac loads/1(Force scale)
  motor params/1 -> Bus Selector3/1
  [system_type] -> isecat1/1
  isecat1/1 -> apply pmac loads/Enable
  system_type/1 -> [system_type]
  [system_type] -> isecat/1
  torques/1 -> [torques]
  [torques] -> apply pmac loads/2(Torques)
  isecat/1 -> EtherCAT Apply Loads/Enable
  [torques] -> EtherCAT Apply Loads/1

== system Bruening_4t_showshuffle/DataLogging/compare encoders ==
  Bus Selector4 : BusSelector  OutputSignals=Robot1.a1_link_angles,Robot2.a2_link_angles
  Bus Selector5 : BusSelector  OutputSignals=robot1.a1_link_angles,robot2.a2_link_angles
  Mux : Mux  Inputs=2
  Mux1 : Mux  Inputs=2
  delta : MATLAB Function  TreatAsAtomicUnit=on
  encoder deltas : Outport
  wires:
  [KINdata_bus] -> Bus Selector4/1
  [primary_encoder_data_bus] -> Bus Selector5/1
  Bus Selector4/1 -> Mux/1  "<a1_link_angles>"
  Bus Selector4/2 -> Mux/2  "<a2_link_angles>"
  Bus Selector5/1 -> Mux1/1  "<a1_link_angles>"
  Bus Selector5/2 -> Mux1/2  "<a2_link_angles>"
  Mux/1 -> delta/1(secondaryEncAngles)
  Mux1/1 -> delta/2(primaryEncAngles)
  delta/1(deltas) -> encoder deltas/1

== system Bruening_4t_showshuffle/DataLogging/Network Transfer Subsystem/Data Packing Subsystem ==
  note: This subsystem packs data frames to create the data portion of the UDP packets, and sets its strobe output high to indicate when a
      | new chunk of packed data is ready. The number of frames per packet is determined to be the smaller of floor(300/width of signal)
      | and 6, as i) we aim at a maximum size of around 1200 to keep it well below the MTU (300x4 bytes per single), and ii) the hardwired
      | delay structure below stores at most 6 frames before adding empty zeros. A size 300 output is always created, as having an undefined
      | port width causes Simulink problems.
  data_frame : Inport
  Constant : Constant  Value=0*[1:300]  OutDataTypeStr=single
  Constant1 : Constant  Value=0
  Counter : Subsystem
  Data Type Conversion : DataTypeConversion  OutDataTypeStr=single  SaturateOnIntegerOverflow=on  RndMeth=Zero
  Ideal Frames Per Packet : Fcn  Expr=floor(300/u(1))
  Math Function : Math  Operator=mod  SaturateOnIntegerOverflow=on
  Max Frames Per Packet : Constant  Value=6
  MinMax : MinMax  Inputs=2
  Mux : Mux  Inputs=7
  Product : Product  RndMeth=Zero
  Relational Operator : RelationalOperator  Operator===  OutDataTypeStr=boolean
  Selector : Selector  IndexMode=Zero-based  IndexOptions=Starting index (port)  Indices=[1:300]  OutputSizes=[([([([([(300)])])])])]
  Subtract : Sum  Inputs=+-
  Width : Width
  t-{1..5} (5 alike) : Memory  InheritSampleTime=on
  daq_packet_strobe : Outport
  packed_data : Outport  Port=2
  wires:
  Ideal Frames Per Packet/1 -> MinMax/2
  Width/1 -> Ideal Frames Per Packet/1, Product/1
  Product/1 -> Selector/2
  Subtract/1 -> Product/2
  Max Frames Per Packet/1 -> MinMax/1, Subtract/1
  MinMax/1 -> Subtract/2, Math Function/2
  Constant/1 -> Mux/7
  Selector/1 -> packed_data/1
  Mux/1 -> Selector/1
  t-5/1 -> Mux/1
  Data Type Conversion/1 -> Mux/6, t-1/1
  t-3/1 -> Mux/3, t-4/1
  t-4/1 -> Mux/2, t-5/1
  t-2/1 -> Mux/4, t-3/1
  t-1/1 -> Mux/5, t-2/1
  Math Function/1 -> Relational Operator/2
  Constant1/1 -> Relational Operator/1
  Relational Operator/1 -> daq_packet_strobe/1
  Counter/1(Y) -> Math Function/1
  data_frame/1 -> Data Type Conversion/1, Width/1

== system Bruening_4t_showshuffle/DataLogging/Network Transfer Subsystem/UDP Receiver ==
  note: DEX-3274: This is the heart of a fix for problems we have found in the UDP sub-system.
      | This code we derrived from the standard UDP receive blocks. The idea here is that the UDP receive
      | block works more-or-less as normal for UDP receive. The main differences are:
      | 1. This version reads the UDP stack twice each time step. This is to look for bad packets and corruption in the UDP stack
      | 2. If this version detects a problem in the UDP stack a call out is made to UDP Receive Port Reset and no more reading is done until the reset is complete.
      |
      | The UDP Receive Port Reset block closes an open UDP port, then reoopens it. This appears to fix any corruption in the UDP stack for the given port.
      | It is critical that this block runs at a relatively slow speed since the reset can take up to 150 micro seconds.
  Trigger UDP reset : Inport
  Data Type Conversion : DataTypeConversion
  Memory2 : Memory  InheritSampleTime=on
  Rate Transition1 : RateTransition
  Rate Transition2 : RateTransition
  Terminator{3..7} (5 alike) : Terminator
  UDP Receive : S-Function  FunctionName=BKINUDPReceiveRead  Parameters=ipAdd, ipPort, width, sampletime, vblLen  mask(BKIN UDP Receive Read){ipAddress=999.999.999.999, ipPort=0, width=4, vblLen=off, sampletime=BKIN_STEP_TIME}
      mask prompts: ipAddress "Source IP address:"; ipPort "Local (destination) port:"; width "Output port width (number of bytes):"; vblLen "Allow variable length packets"; sampletime "Sample time:"
      mask help:
      | Modified from legacy UDP Receive block.
      | The rationale for modifying was to enable resetting of the UDP Port while running a model.
      | Because resetting can potentially take longer than one clock cycle, the resetting needed to be split off from the reading to allow them to run at different update rates.
      |
      | Click Help for more details.
      mask init:
      | % BKIN - I tried commenting these out, but it causes build errors.
      | mudp('ipPort', 'IP Port');
      | ipAdd = ipAddressFromString(ipAddress);
      mask Help:
      | Used to read UDP packets. Modified from legacy UDP Read Receive. Must be used with BKIN UDP Receive Port Reset block.
      | 
      | <H2>Description </H2>
      | This block reads a UDP packet from an IP address and port specified in the BKIN UDP Receive Port Reset block.
      | <P>
      | If a packet is read, it will read attempt to read a second packet (i.e. to clear out the queue).
      | <P>
      | If a UDP reset trigger is received, it will coordinate a UDP port reset with the BKIN UDP Receive Port Reset block.
      | During the resetting, UDP reads will not occur.
      |  <P>
      | 
      | <B>UDP Reset Trigger: </B> when this input goes to 1 for at least one clock cycle, it will initiate a reset of the UDP port.
      | <P>
      | <B>Port Info: </B> this vector input must come from the BKIN UDP Receive Port Reset block.
      | <P>
      | <B>Data: </B> This output contains the most recent data read from the UDP packet
      | <P>
      | <B>N: </B> This output contains 1 when a UDP packet was read (or if variable length was checked, the length of the packet).
      | It contains -1 if reads are not allowed (i.e. because the port is being reset).
      | It contains 0 if there was no packet to read.
      | It contains -9 if the length specified in the mask of this block is different that what was specified when the port was opened (i.e. via the BKIN UDP Receive Port Reset block).
      | <P>
      | <B>Data 2: </B> This output contains  the most recent data read from the second read UDP packet (if one was read)
      | <P>
      | <B>N 2: </B> This output contains the same information as the output "N", but for the second UDP packet.
      | <P>
      | <B># double reads: </B> This output contains  the number of times that two UDP packets were read in a single time frame since the start of the task.
      | <P>
      | <B>Request UDP Reset: </B> This output should be connected to UDP Reset input of BKIN UDP Receive Port Reset. It will go to 1 when UDP trigger reset is recieved, and it will stay at 1 until an acknowledgement has been received via Port Info
      | <P>
      | 
      | 
      | <H2>Parameters and Dialog Box</H2>
      | <P>
      | <B>Output port width</B> this value must be specified, and must be the same as the associated value on the BKIN UDP Receieve Port Reset Block.
      | <P>
      | <B>Allow variable length packets: </B> This input is left-over from the legacy block. Leave unchecked, as it is has not been tested yet.
      | <P>
      | <B>Sample Time: </B> May be set to a faster update rate than the BKIN UDP Receive Port Reset.
      | <P>
      | 
      | <H2>Related Blocks </H2>
      | BKIN UDP Receive Port Reset<BR>
      mask Display:
      | disp( sprintf('BKIN UDP\nReceive\nBinary\n(%d bytes)', width));
      | port_label('output', 1, 'Data');
      | port_label('output', 2, 'N');
      | port_label('output', 3, 'Data 2');
      | port_label('output', 4, 'N 2');
      | port_label('output', 5, '# double reads');
      | port_label('output', 6, 'Request UDP Reset');
      | port_label('input', 1, 'UDP Reset Trigger');
      | port_label('input', 2, 'Port Info');
  UDP Receive Port Reset : S-Function  FunctionName=BKINUDPReceiveInit  Parameters=ipAdd, ipPort, width, sampletime, vblLen  mask(BKIN UDP Receive Port Reset){ipAddress=192.168.0.1, ipPort=50001, width=4, vblLen=off, sampletime=0.001}
      mask prompts: ipAddress "Source IP address:"; ipPort "Local (destination) port:"; width "Output port width (number of bytes):"; vblLen "Allow variable length packets"; sampletime "Sample time:"
      mask help:
      | Modified from legacy UDP Receive block.
      | The rationale for modifying was to enable resetting of the UDP Port while running a model.
      | Because resetting can potentially take longer than one clock cycle, the resetting needed to be split off from the reading to allow them to run at different update rates.
      |
      | Click Help for more details.
      mask init:
      | mudp('ipPort', 'IP Port');
      | ipAdd = ipAddressFromString(ipAddress);
      mask Help:
      | Used to read UDP packets. Modified from legacy UDP Read Receive. Must be used with BKIN UDP Receive Read block.
      | 
      | <H2>Description </H2>
      | This block initializes, closes, and can reset a UDP Receive port.
      | <P>
      | 
      | <B>UDP Reset: </B> this input must come from a BKIN UDP Receive Read block. When this input goes to 1, it will initiate a reset of the UDP port. It will send an acknowledgement that a reset is occuring as part of the output Port Info
      | <P>
      | <B># Resets: </B> This output contains the number of times that the UDP port has been reset.
      | <P>
      | <B>Port Info: </B> this vector output must go to the BKIN UDP Receive Read block. It contains information related to the port ID, the length of the expected packet and the status of the port reset.
      | <P>
      | 
      | <H2>Parameters and Dialog Box</H2>
      | <P>
      | <B>Source IP Address</B> in the form of xxx.xxx.xxx.xxx
      | <P>
      | <B>Local (destination) port</B> the port to be used.
      | <P>
      | <B>Output port width</B> this value must be specified, and must be the same as the associated value on the BKIN UDP Receieve Read Block.
      | <P>
      | <B>Sample time: </B> May be set to a slower update rate than the BKIN UDP Receive Read.
      | <P>
      | 
      | <H2>Related Blocks </H2>
      | BKIN UDP Receive Read<BR>
      mask Display:
      | disp( sprintf('BKIN UDP\nReceive\nPort Reset\n  (%d bytes)', width));
      | port_label('output', 1, '# Resets');
      | port_label('output', 2, 'Port Info');
      | port_label('input', 1, 'UDP Reset');
  Unpack : xpcobsoletelib/Utilities/Unpack   dimensions={[1]}  datatypes={'single'}  byteAlign=1
  ACK_ID : Outport
  wires:
  UDP Receive/1 -> Unpack/1  "Data"
  UDP Receive/4 -> Terminator4/1  "Pckt_Recd 2"
  UDP Receive/3 -> Terminator3/1  "Data 2"
  UDP Receive Port Reset/2 -> Rate Transition2/1
  Memory2/1 -> UDP Receive/1  "trigger"
  Rate Transition2/1 -> UDP Receive/2
  Rate Transition1/1 -> UDP Receive Port Reset/1  "Rqst UDP Reset"
  UDP Receive Port Reset/1 -> Terminator6/1  "# UDP Resets"
  UDP Receive/6 -> Rate Transition1/1
  UDP Receive/5 -> Terminator5/1  "# double reads"
  UDP Receive/2 -> Terminator7/1  "Pckt_Recd"
  Unpack/1 -> Data Type Conversion/1
  Data Type Conversion/1 -> ACK_ID/1
  Trigger UDP reset/1 -> Memory2/1

== system Bruening_4t_showshuffle/DataLogging/Network Transfer Subsystem/UDP Send Subsystem ==
  packet_data : Inport
  Trigger : TriggerPort  TriggerType=function-call
  Counter Free-Running : simulink/Sources/Counter Free-Running  NumBits=32  tsamp=-1
  Pack : xpcobsoletelib/Utilities/Pack   datatypes={'single'}  byteAlign=1
  Send : xpcrtudplib/Legacy UDP/Send   ipAddress=192.168.0.1  ipPort=50000  localPort=50000  vblLen=off  sampletime=-1
  Total Packets Sent : DataTypeConversion  OutDataTypeStr=double  SaturateOnIntegerOverflow=on  RndMeth=Zero
  total_packets_sent : Outport  InitialOutput=0
  wires:
  packet_data/1 -> Pack/1
  Pack/1 -> Send/1
  Counter Free-Running/1 -> Total Packets Sent/1
  Total Packets Sent/1 -> total_packets_sent/1
